simulink model "sl_mobile_vs2"  (R2015b)
settings: Solver=ode45  StartTime=0.0  StopTime=10  RelTol=1e-3
InitFcn:
  | camera = CentralCamera('default', 'name', 'mobile_vs', 'focal', 0.002);
  | T_vc = transl(0.2, 0.1, 0.3)*troty(pi/2)*trotz(-pi/2); %*trotx(-pi/4);
  | P = [0 0; 1 -1; 2 2];
  | pstar = camera.project(P, 'Tcam', transl(-2, 0, 0)*T_vc);
undefined symbols (not defined in the file): DiscIntNeverNeededParam, transl, trotz
libraries: roblocks x5, simulink x1
settings Model: ExtModeTrigMode=oneshot  ExtModeArmWhenConnect=off  Creator=pic  LastModifiedBy=corkep
settings DataIOCC: LimitDataPoints=off  SaveFormat=Structure  SignalLoggingSaveFormat=ModelDataLogs  ReturnWorkspaceOutputs=on
settings OptimizationCC: BlockReduction=off  BooleanDataType=off  ExpressionDepthLimit=2147483647  InitFltsAndDblsToZero=on
settings DebuggingCC: SaveWithParameterizedLinksMsg=none  UnderspecifiedInitializationDetection=Classic  MergeDetectMultiDrivingBlocksExec=none  SignalResolutionControl=TryResolveAllWithWarning  MultiTaskDSMMsg=warning  MultiTaskCondExecSysMsg=none  FcnCallInpInsideContextMsg=UseLocalSettings  StateNameClashWarn=warning
settings HardwareCC: ProdBitPerPointer=32  ProdLargestAtomicFloat=None  ProdIntDivRoundTo=Undefined  ProdEndianess=Unspecified  ProdWordSize=32  ProdHWDeviceType=32-bit Generic  TargetUnknown=on
settings GRTTargetCC: ModelReferenceCompliant=off  CompOptLevelCompliant=off  GeneratePreprocessorConditionals=Disable all  CombineOutputUpdateFcns=off  MatFileLogging=off  GRTInterface=on
settings ConfigComp: CovModelRefEnable=Off  CovSFcnEnable=off

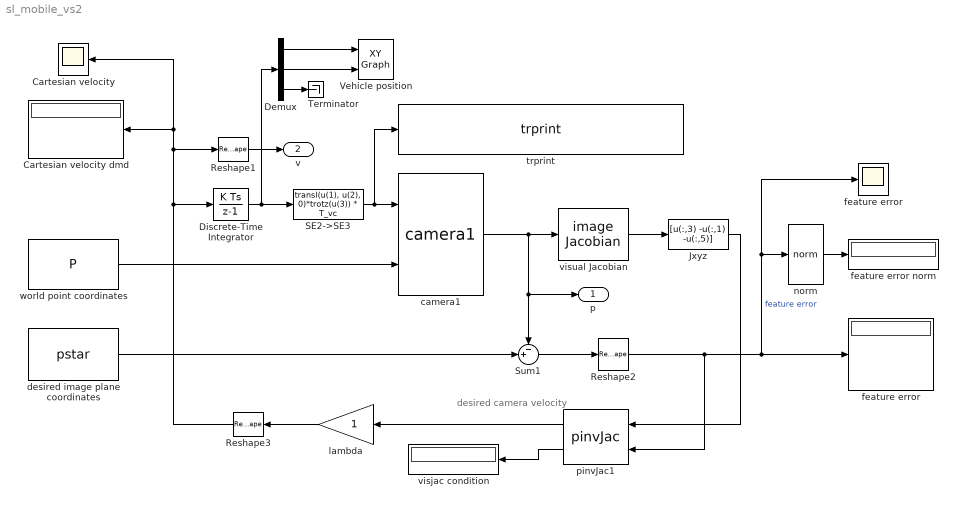
== system sl_mobile_vs2 ==
  note: desired camera velocity
  Cartesian velocity : Scope
  Cartesian velocity dmd : Display
      settings: Format=bank
  Demux : Demux  Outputs=3
  Discrete-Time Integrator : DiscreteIntegrator  InitialCondition=[-8 2 0.3]'  SampleTime=0.02  ICPrevOutput=DiscIntNeverNeededParam  ICPrevScaledInput=DiscIntNeverNeededParam
  Jxyz : MATLABFcn  MATLABFcn=[u(:,3) -u(:,1) -u(:,5)]  Output1D=off
  Reshape1 : Reshape  OutputDimensions=6
  Reshape2 : Reshape  OutputDimensions=6
  Reshape3 : Reshape  OutputDimensions=6
  SE2->SE3 : MATLABFcn  MATLABFcn=transl(u(1), u(2), 0)*trotz(u(3)) * T_vc  Output1D=off
  Sum1 : Sum  Inputs=-+|  SaturateOnIntegerOverflow=on  InputSameDT=on  OutDataTypeStr=Inherit: Same as first input
  Terminator : Terminator
  Vehicle position : simulink/Sinks/XY Graph  xmin=-10  xmax=10  ymin=-10  ymax=10  st=-1
  camera1 : roblocks/Vision/camera1  cam=camera
  desired image plane coordinates : Constant  Value=pstar  VectorParams1D=off
  feature error : Display
      settings: Format=bank
  feature error norm : Display
  "feature error " : Scope
  lambda : Gain  SaturateOnIntegerOverflow=on  OutDataTypeStr=Inherit: Same as input  ParamDataTypeStr=Inherit: Same as input
  norm : roblocks/Toolbox/norm  SystemSampleTime=-1
  pinvJac1 : roblocks/Toolbox/pinvJac
  trprint : roblocks/Toolbox/trprint  options={'bingo'}
      link override S-Function: Parameters=options
  visjac condition : Display
  visual Jacobian : roblocks/Vision/image Jacobian  cam=camera  z=3
  world point coordinates : Constant  Value=P  VectorParams1D=off
  p : Outport
  v : Outport  Port=2
  wires:
  Sum1/1 -> Reshape2/1
  desired image plane coordinates/1 -> Sum1/2
  Reshape2/1 -> "feature error "/1, norm/1, feature error/1, pinvJac1/2  "feature error"
  pinvJac1/2 -> visjac condition/1
  pinvJac1/1 -> lambda/1
  visual Jacobian/1 -> Jxyz/1
  lambda/1 -> Reshape3/1
  Reshape1/1 -> v/1
  camera1/1 -> Sum1/1, p/1, visual Jacobian/1
  world point coordinates/1 -> camera1/2
  norm/1 -> feature error norm/1
  Discrete-Time Integrator/1 -> SE2->SE3/1, Demux/1
  Demux/1 -> Vehicle position/1
  Demux/2 -> Vehicle position/2
  Jxyz/1 -> pinvJac1/1
  SE2->SE3/1 -> trprint/1, camera1/1
  Demux/3 -> Terminator/1
  Reshape3/1 -> Cartesian velocity/1, Cartesian velocity dmd/1, Reshape1/1, Discrete-Time Integrator/1
